simulink model "Test7"  (R2021b)
settings: Solver=FixedStepAuto  StartTime=0.0  StopTime=Inf  RelTol=1e-3  EnableMultiTasking=on
undefined symbols (not defined in the file): magnitude
libraries: arduinolib x6
settings Model: ExtModeTrigDuration=2  Creator=diego  LastModifiedBy=diego
settings OptimizationCC: EnhancedBackFolding=on  PassReuseOutputArgsAs=Individual arguments  ZeroExternalMemoryAtStartup=off  ZeroInternalMemoryAtStartup=off  MaxStackSize=64  OptimizeBlockOrder=speed  DifferentSizesBufferReuse=on  EfficientTunableParamExpr=on
settings DebuggingCC: ParameterTunabilityLossMsg=error
settings HardwareCC: ProdBitPerInt=16  ProdBitPerPointer=16  ProdBitPerSizeT=16  ProdBitPerPtrDiffT=16  ProdLargestAtomicFloat=None  ProdWordSize=8  ProdHWDeviceType=Atmel->AVR
settings SFSimCC: MATLABDynamicMemAlloc=off
settings RTWCC: Description=Embedded Coder  SystemTargetFile=ert.tlc  HardwareBoard=Arduino Uno  TemplateMakefile=ert_default_tmf  Toolchain=Arduino AVR  BuildConfiguration=Faster Runs
settings CodeAppCC: ForceParamTrailComments=on  IgnoreCustomStorageClasses=off  OperatorAnnotations=on  SimulinkDataObjDesc=on  SFDataObjDesc=on  InsertBlockDesc=on
settings ERTTargetCC: SupportContinuousTime=on  SupportVariableSizeSignals=on  ExtModeTransport=3  ExtModeStaticAlloc=on  ExtModeStaticAllocSize=250  ExtModeMexFile=ext_xcp  ExtModeIntrfLevel=Level2 - Open

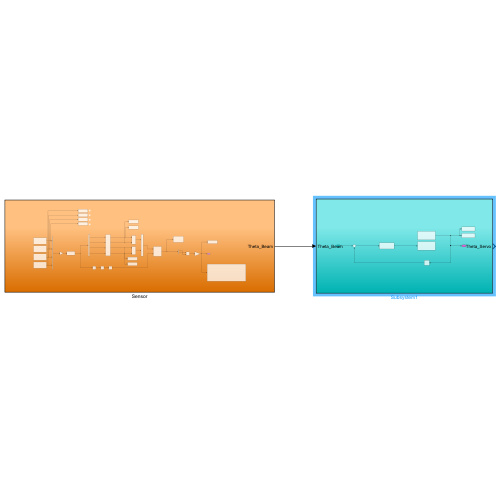
[thumbnail: Simulink's stored preview of the top-level diagram]
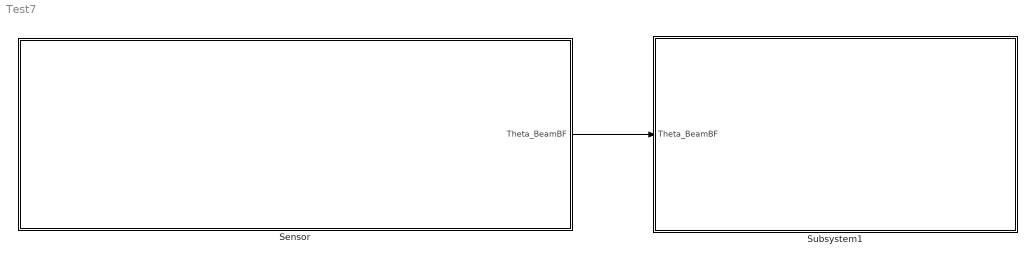
== system Test7 ==
  Sensor : Subsystem
  Subsystem1 : Subsystem
  wires:
  Sensor/1(Theta_BeamBF) -> Subsystem1/1(Theta_BeamBF)

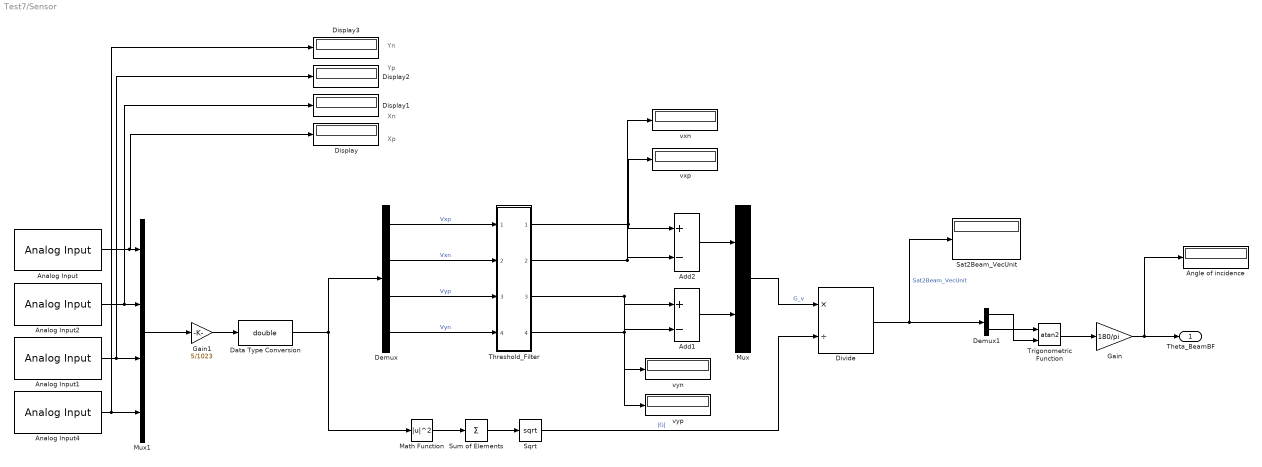
== system Test7/Sensor ==
  note: Yn
  note: Yp
  note: Xn
  note: Xp
  Add1 : Sum  Inputs=+|-
  Add2 : Sum  Inputs=+|-
  Analog Input : arduinolib/Analog Input  pinNumber=0  ReadResultsOnly=off  ConversionTriggerSource=Software  ExternalTriggerType=uint32( 0 )  OutputDataType=uint16  EnableConversionCompleteNotify=off  EnableOuputStatus=off  SampleTime=-1  blockPlatform=arduino
  Analog Input1 : arduinolib/Analog Input  pinNumber=2  ReadResultsOnly=off  ConversionTriggerSource=Software  ExternalTriggerType=uint32( 0 )  OutputDataType=uint16  EnableConversionCompleteNotify=off  EnableOuputStatus=off  SampleTime=-1  blockPlatform=arduino
  Analog Input2 : arduinolib/Analog Input  pinNumber=1  ReadResultsOnly=off  ConversionTriggerSource=Software  ExternalTriggerType=uint32( 0 )  OutputDataType=uint16  EnableConversionCompleteNotify=off  EnableOuputStatus=off  SampleTime=-1  blockPlatform=arduino
  Analog Input4 : arduinolib/Analog Input  pinNumber=3  ReadResultsOnly=off  ConversionTriggerSource=Software  ExternalTriggerType=uint32( 0 )  OutputDataType=uint16  EnableConversionCompleteNotify=off  EnableOuputStatus=off  SampleTime=-1  blockPlatform=arduino
  Angle of incidence : Display
  Data Type Conversion : DataTypeConversion  OutDataTypeStr=double
  Demux : Demux
  Demux1 : Demux  Outputs=2
  Display{,1..3} (4 alike) : Display
  Divide : Product  Inputs=*/
  Gain : Gain  Gain=180/pi
  Gain1 : Gain  Gain=5/1023
  Math Function : Math  Operator=magnitude^2  OutputSignalType=real  SaturateOnIntegerOverflow=on
  Mux : Mux  Inputs=2
  Mux1 : Mux
  Sat2Beam_VecUnit : Display
  Sqrt : Sqrt  SaturateOnIntegerOverflow=on
  Sum of Elements : Sum  Inputs=+
  Threshold_Filter : Subsystem
  Trigonometric Function : Trigonometry  Operator=atan2
  vxn : Display
  vxp : Display
  vyn : Display
  vyp : Display
  Theta_BeamBF : Outport
  wires:
  Sqrt/1 -> Divide/2  "|G|"
  Threshold_Filter/1(Out1) -> vxp/1, Add2/1
  Threshold_Filter/2(Out2) -> Add2/2, vxn/1
  Data Type Conversion/1 -> Math Function/1, Demux/1
  Analog Input1/1 -> Mux1/3, Display2/1
  Threshold_Filter/4(Out4) -> vyn/1, Add1/2
  Threshold_Filter/3(Out3) -> vyp/1, Add1/1
  Analog Input4/1 -> Mux1/4, Display3/1
  Add1/1 -> Mux/2
  Analog Input/1 -> Display/1, Mux1/1
  Sum of Elements/1 -> Sqrt/1
  Demux/2 -> Threshold_Filter/2(Vxn)  "Vxn"
  Demux/4 -> Threshold_Filter/4(Vyn)  "Vyn"
  Demux/3 -> Threshold_Filter/3(Vyp)  "Vyp"
  Analog Input2/1 -> Display1/1, Mux1/2
  Add2/1 -> Mux/1
  Mux/1 -> Divide/1  "G_v"
  Gain1/1 -> Data Type Conversion/1
  Math Function/1 -> Sum of Elements/1
  Mux1/1 -> Gain1/1
  Demux/1 -> Threshold_Filter/1(Vxp)  "Vxp"
  Gain/1 -> Angle of incidence/1, Theta_BeamBF/1
  Demux1/1 -> Trigonometric Function/2
  Trigonometric Function/1 -> Gain/1
  Divide/1 -> Demux1/1, Sat2Beam_VecUnit/1  "Sat2Beam_VecUnit"
  Demux1/2 -> Trigonometric Function/1

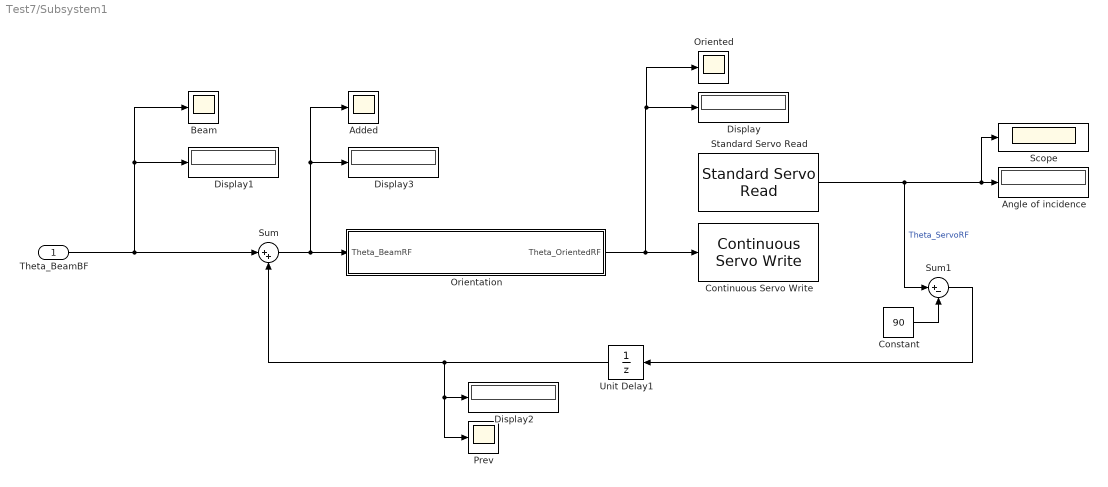
== system Test7/Subsystem1 ==
  Theta_BeamBF : Inport
  Added : Scope
  Angle of incidence : Display
  Beam : Scope
  Constant : Constant  Value=90
  Continuous Servo Write : arduinolib/Continuous Servo Write  pinNumber=9  ServoIndex=0  blockPlatform=ARDUINO
      settings: SourceProductBaseCode=ARDUINO
  Display{,1..3} (4 alike) : Display
  Orientation : Subsystem
  Oriented : Scope
  Prev : Scope
  Scope : Scope
  Standard Servo Read : arduinolib/Standard Servo Read  pinNumber=9  SampleTime=0.1  ServoIndex=0  blockPlatform=ARDUINO
      settings: SourceProductBaseCode=ARDUINO
  Sum : Sum  Inputs=|++
  Sum1 : Sum  Inputs=|+-
  Unit Delay1 : UnitDelay  SampleTime=-1  HasFrameUpgradeWarning=on
  wires:
  Sum/1 -> Added/1, Display3/1, Orientation/1(Theta_BeamRF)
  Standard Servo Read/1 -> Scope/1, Angle of incidence/1, Sum1/1  "Theta_ServoRF"
  Unit Delay1/1 -> Prev/1, Display2/1, Sum/2
  Theta_BeamBF/1 -> Beam/1, Display1/1, Sum/1
  Orientation/1(Theta_OrientedRF) -> Continuous Servo Write/1, Oriented/1, Display/1
  Sum1/1 -> Unit Delay1/1
  Constant/1 -> Sum1/2

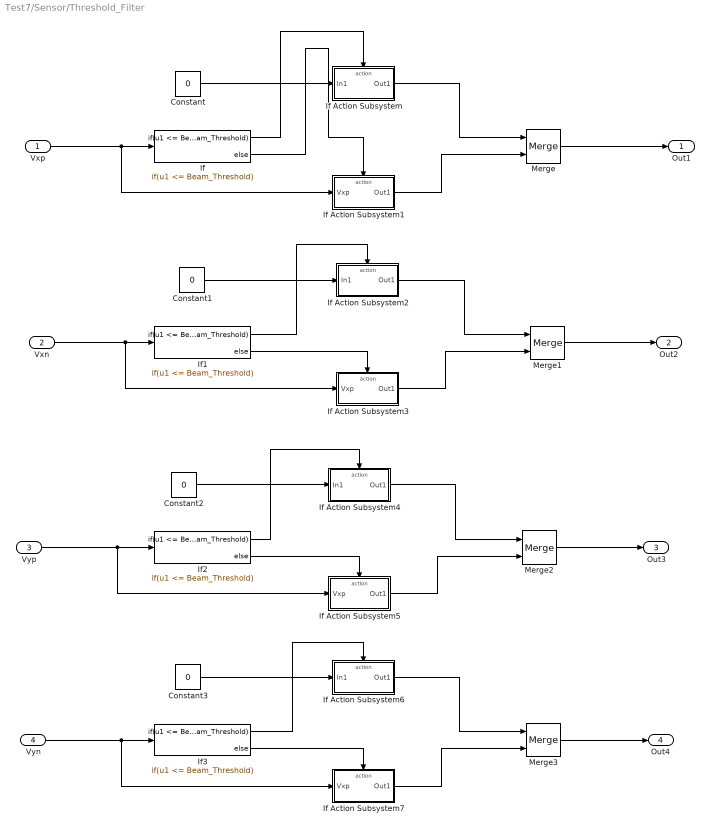
== system Test7/Sensor/Threshold_Filter ==
  Vxp : Inport
  Vxn : Inport  Port=2
  Vyp : Inport  Port=3
  Vyn : Inport  Port=4
  Constant{,1..3} (4 alike) : Constant  Value=0
  If{,1..3} (4 alike) : If  IfExpression=u1 <= Beam_Threshold
  If Action Subsystem : Subsystem  TreatAsAtomicUnit=on
  If Action Subsystem1 : Subsystem  TreatAsAtomicUnit=on
  If Action Subsystem2 : Subsystem  TreatAsAtomicUnit=on
  If Action Subsystem3 : Subsystem  TreatAsAtomicUnit=on
  If Action Subsystem4 : Subsystem  TreatAsAtomicUnit=on
  If Action Subsystem5 : Subsystem  TreatAsAtomicUnit=on
  If Action Subsystem6 : Subsystem  TreatAsAtomicUnit=on
  If Action Subsystem7 : Subsystem  TreatAsAtomicUnit=on
  Merge{,1..3} (4 alike) : Merge
  Out1 : Outport
  Out2 : Outport  Port=2
  Out3 : Outport  Port=3
  Out4 : Outport  Port=4
  wires:
  Vxp/1 -> If Action Subsystem1/1(Vxp), If/1
  If/1 -> If Action Subsystem/Action
  If Action Subsystem/1(Out1) -> Merge/1
  If/2 -> If Action Subsystem1/Action
  If Action Subsystem1/1(Out1) -> Merge/2
  Merge/1 -> Out1/1
  Constant/1 -> If Action Subsystem/1(In1)
  If Action Subsystem3/1(Out1) -> Merge1/2
  Constant1/1 -> If Action Subsystem2/1(In1)
  If1/1 -> If Action Subsystem2/Action
  Vxn/1 -> If1/1, If Action Subsystem3/1(Vxp)
  If Action Subsystem2/1(Out1) -> Merge1/1
  If1/2 -> If Action Subsystem3/Action
  Merge1/1 -> Out2/1
  Vyp/1 -> If2/1, If Action Subsystem5/1(Vxp)
  If2/2 -> If Action Subsystem5/Action
  If2/1 -> If Action Subsystem4/Action
  If Action Subsystem4/1(Out1) -> Merge2/1
  If Action Subsystem5/1(Out1) -> Merge2/2
  Constant2/1 -> If Action Subsystem4/1(In1)
  Merge2/1 -> Out3/1
  Vyn/1 -> If3/1, If Action Subsystem7/1(Vxp)
  Merge3/1 -> Out4/1
  If Action Subsystem7/1(Out1) -> Merge3/2
  If3/2 -> If Action Subsystem7/Action
  If Action Subsystem6/1(Out1) -> Merge3/1
  Constant3/1 -> If Action Subsystem6/1(In1)
  If3/1 -> If Action Subsystem6/Action

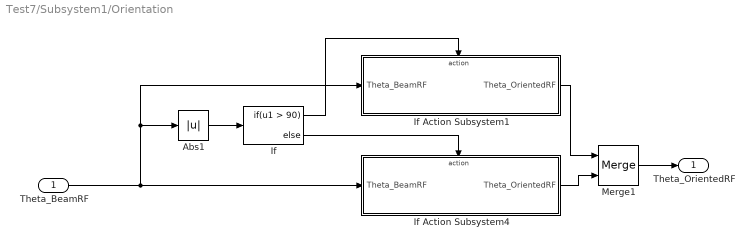
== system Test7/Subsystem1/Orientation ==
  Theta_BeamRF : Inport
  Abs1 : Abs
  If : If  IfExpression=u1 > 90
  If Action Subsystem1 : Subsystem  TreatAsAtomicUnit=on
  If Action Subsystem4 : Subsystem  TreatAsAtomicUnit=on
  Merge1 : Merge
  Theta_OrientedRF : Outport
  wires:
  If Action Subsystem1/1(Theta_OrientedRF) -> Merge1/1
  Merge1/1 -> Theta_OrientedRF/1
  If/2 -> If Action Subsystem4/Action
  If/1 -> If Action Subsystem1/Action
  Abs1/1 -> If/1
  Theta_BeamRF/1 -> If Action Subsystem1/1(Theta_BeamRF), Abs1/1, If Action Subsystem4/1(Theta_BeamRF)
  If Action Subsystem4/1(Theta_OrientedRF) -> Merge1/2

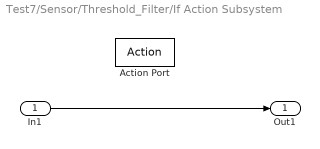
== system Test7/Sensor/Threshold_Filter/If Action Subsystem ==
  In1 : Inport
  Action Port : ActionPort  ActionPortLabel=if(u1 <= Beam_Threshold)
  Out1 : Outport
  wires:
  In1/1 -> Out1/1

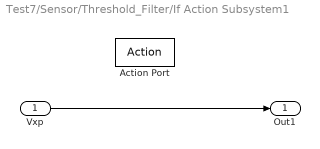
== system Test7/Sensor/Threshold_Filter/If Action Subsystem1 ==
  Vxp : Inport
  Action Port : ActionPort  ActionPortLabel=else
  Out1 : Outport
  wires:
  Vxp/1 -> Out1/1

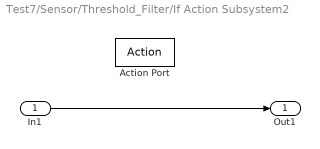
== system Test7/Sensor/Threshold_Filter/If Action Subsystem2 ==
  In1 : Inport
  Action Port : ActionPort  ActionPortLabel=if(u1 <= Beam_Threshold)
  Out1 : Outport
  wires:
  In1/1 -> Out1/1

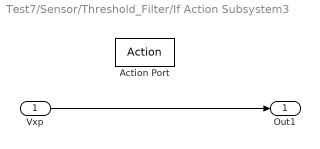
== system Test7/Sensor/Threshold_Filter/If Action Subsystem3 ==
  Vxp : Inport
  Action Port : ActionPort  ActionPortLabel=else
  Out1 : Outport
  wires:
  Vxp/1 -> Out1/1

== system Test7/Sensor/Threshold_Filter/If Action Subsystem4 ==
  In1 : Inport
  Action Port : ActionPort  ActionPortLabel=if(u1 <= Beam_Threshold)
  Out1 : Outport
  wires:
  In1/1 -> Out1/1

== system Test7/Sensor/Threshold_Filter/If Action Subsystem5 ==
  Vxp : Inport
  Action Port : ActionPort  ActionPortLabel=else
  Out1 : Outport
  wires:
  Vxp/1 -> Out1/1

== system Test7/Sensor/Threshold_Filter/If Action Subsystem6 ==
  In1 : Inport
  Action Port : ActionPort  ActionPortLabel=if(u1 <= Beam_Threshold)
  Out1 : Outport
  wires:
  In1/1 -> Out1/1

== system Test7/Sensor/Threshold_Filter/If Action Subsystem7 ==
  Vxp : Inport
  Action Port : ActionPort  ActionPortLabel=else
  Out1 : Outport
  wires:
  Vxp/1 -> Out1/1

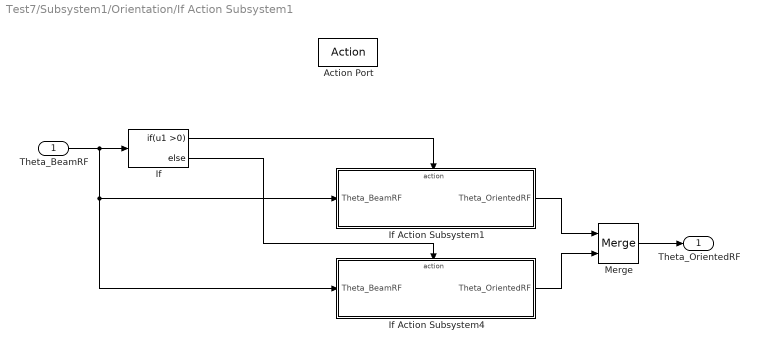
== system Test7/Subsystem1/Orientation/If Action Subsystem1 ==
  Theta_BeamRF : Inport
  Action Port : ActionPort  ActionPortLabel=if(u1 > 90)
  If : If  IfExpression=u1 >0
  If Action Subsystem1 : Subsystem  TreatAsAtomicUnit=on
  If Action Subsystem4 : Subsystem  TreatAsAtomicUnit=on
  Merge : Merge
  Theta_OrientedRF : Outport
  wires:
  Theta_BeamRF/1 -> If Action Subsystem4/1(Theta_BeamRF), If Action Subsystem1/1(Theta_BeamRF), If/1
  If/1 -> If Action Subsystem1/Action
  If/2 -> If Action Subsystem4/Action
  If Action Subsystem1/1(Theta_OrientedRF) -> Merge/1
  If Action Subsystem4/1(Theta_OrientedRF) -> Merge/2
  Merge/1 -> Theta_OrientedRF/1

== system Test7/Subsystem1/Orientation/If Action Subsystem4 ==
  Theta_BeamRF : Inport
  Action Port : ActionPort  ActionPortLabel=else
  Theta_OrientedRF : Outport
  wires:
  Theta_BeamRF/1 -> Theta_OrientedRF/1

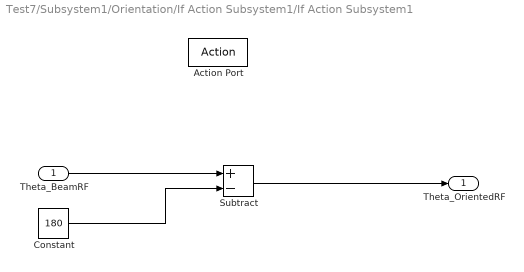
== system Test7/Subsystem1/Orientation/If Action Subsystem1/If Action Subsystem1 ==
  Theta_BeamRF : Inport
  Action Port : ActionPort  ActionPortLabel=if(u1 >0)
  Constant : Constant  Value=180
  Subtract : Sum  Inputs=+-
  Theta_OrientedRF : Outport
  wires:
  Subtract/1 -> Theta_OrientedRF/1
  Theta_BeamRF/1 -> Subtract/1
  Constant/1 -> Subtract/2

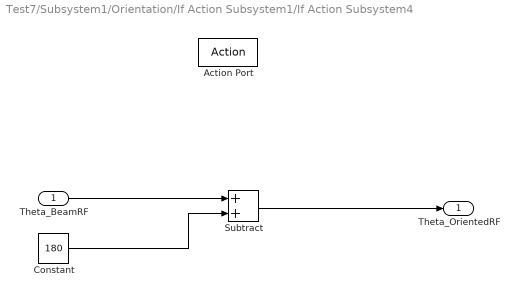
== system Test7/Subsystem1/Orientation/If Action Subsystem1/If Action Subsystem4 ==
  Theta_BeamRF : Inport
  Action Port : ActionPort  ActionPortLabel=else
  Constant : Constant  Value=180
  Subtract : Sum
  Theta_OrientedRF : Outport
  wires:
  Theta_BeamRF/1 -> Subtract/1
  Constant/1 -> Subtract/2
  Subtract/1 -> Theta_OrientedRF/1
